simulink model "Example_Hydraulic_ValveThermostatic2"  (R2013b)
settings: Solver=ode45  StartTime=0.0  StopTime=3*3600  RelTol=1e-3
libraries: carnot x4, simulink x1
settings Model: Creator=drhf  LastModifiedBy=drhf
settings OptimizationCC: ExpressionDepthLimit=2147483647
settings DebuggingCC: StateNameClashWarn=warning
settings GRTTargetCC: CombineOutputUpdateFcns=off  GRTInterface=on

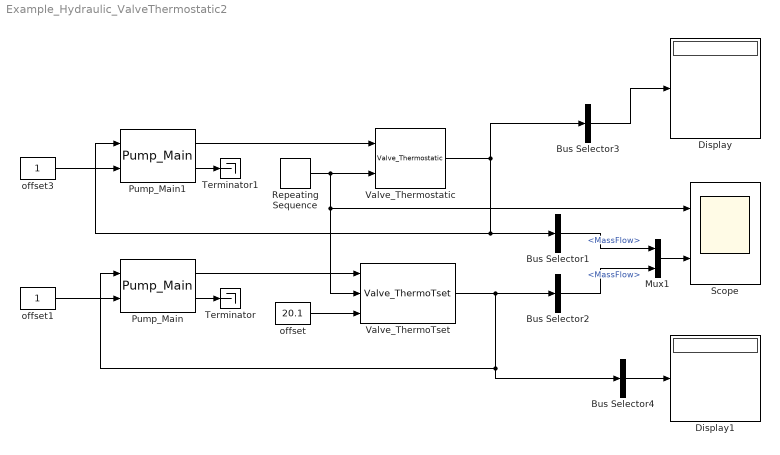
== system Example_Hydraulic_ValveThermostatic2 ==
  Bus Selector1 : BusSelector  OutputSignals=MassFlow
  Bus Selector2 : BusSelector  OutputSignals=MassFlow
  Bus Selector3 : BusSelector  OutputSignals=DPConstant,DPLinear,DPQuadratic  OutputAsBus=on
  Bus Selector4 : BusSelector  OutputSignals=DPConstant,DPLinear,DPQuadratic  OutputAsBus=on
  Display : Display
  Display1 : Display
  Mux1 : Mux  Inputs=2
  Pump_Main : carnot/Hydraulics/Pump_Main  a0=2.7e4  a1=-1.2e4  a2=0%-3e-3  dia=0.025  t1=5  p0=3e5  IDchk=off  fluid_id=Water  mix=0  ua=1  mcp=500  tamb=20
  Pump_Main1 : carnot/Hydraulics/Pump_Main  a0=2.7e4  a1=-1.2e4  a2=0%-3e-3  dia=0.025  t1=5  p0=3e5  IDchk=off  fluid_id=Water  mix=0  ua=1  mcp=500  tamb=20
  Repeating Sequence : simulink/Sources/Repeating Sequence  rep_seq_t=[0 1 2]*3600  rep_seq_y=[19 21 19]
  Scope : Scope  NumInputPorts=2
      settings: YMin=-5~-5  YMax=5~5
  Terminator : Terminator
  Terminator1 : Terminator
  Valve_ThermoTset : carnot/Hydraulics/Valve_ThermoTset  p=3  op=0.5  bl=0.1  ts=10  dia=0.02  vpos=[0 0.1 1]  vqua=[1e6 1e6 1]
  Valve_Thermostatic : carnot/Hydraulics/Valve_Thermostatic  Tset=20  prange=3  op=0.5  bl=0.1  ts=10  dia=0.02  vpos=[0 0.1 1]  vqua=[1e6 1e6 1]
  offset : Constant  Value=20.1
  offset1 : Constant
  offset3 : Constant
  wires:
  offset/1 -> Valve_ThermoTset/3
  Pump_Main/1 -> Valve_ThermoTset/1
  Valve_ThermoTset/1 -> Bus Selector4/1, Pump_Main/1, Bus Selector2/1
  offset1/1 -> Pump_Main/2
  Pump_Main1/1 -> Valve_Thermostatic/1
  Valve_Thermostatic/1 -> Pump_Main1/1, Bus Selector1/1, Bus Selector3/1
  offset3/1 -> Pump_Main1/2
  Pump_Main/2 -> Terminator/1
  Pump_Main1/2 -> Terminator1/1
  Repeating Sequence/1 -> Valve_Thermostatic/2, Valve_ThermoTset/2, Scope/1
  Mux1/1 -> Scope/2
  Bus Selector1/1 -> Mux1/1  "<MassFlow>"
  Bus Selector2/1 -> Mux1/2  "<MassFlow>"
  Bus Selector3/1 -> Display/1
  Bus Selector4/1 -> Display1/1
